simulink model "modelsim_cosimulation"  (R2021b)
settings: Solver=FixedStepDiscrete  StartTime=0.0  StopTime=4402*Ts  RelTol=1e-3
model workspace (MAT data in the model file):
  ErrMarginBits = 4
  Ts = 10
  inputdata.time = [0 10 20 30 40 50 60 70 80 90 100 110 ... (4402 elements, 4402x1)]
  inputdata.signals.values = embedded.fi
  inputdata.signals.values.DataType = 'Fixed'
  inputdata.signals.values.Scaling = 'BinaryPoint'
  inputdata.signals.values.Signed = 1
  inputdata.signals.values.WordLength = 12
  inputdata.signals.values.FixedExponent = 0
  inputdata.signals.values.SlopeAdjustmentFactor = 1
  inputdata.signals.values.Bias = 0
  inputdata.signals.values.DataTypeOverride = 'Inherit'
  inputdata.signals.values.intarray = [1 0 0 0 0 0 0 0 0 0 0 0 ... (4402 elements, 4402x1)]
  inputdata.signals.values.noverflows = 0
  inputdata.signals.values.nunderflows = 0
  inputdata.signals.values.maxlog = -1.79769313486e+308
  inputdata.signals.values.minlog = 1.79769313486e+308
  inputdata.signals.values.RoundingMethod = 'Round'
  inputdata.signals.values.OverflowAction = 'Saturate'
  inputdata.signals.values.ProductMode = 'FullPrecision'
  inputdata.signals.values.SumMode = 'FullPrecision'
  inputdata.signals.values.ProductWordLength = 32
  inputdata.signals.values.SumWordLength = 32
  inputdata.signals.values.MaxProductWordLength = 65535
  inputdata.signals.values.MaxSumWordLength = 65535
  inputdata.signals.values.ProductFractionLength = 30
  inputdata.signals.values.ProductFixedExponent = -30
  inputdata.signals.values.ProductSlope = 9.31322574615e-10
  inputdata.signals.values.ProductSlopeAdjustmentFactor = 1
  inputdata.signals.values.ProductBias = 0
  inputdata.signals.values.SumFractionLength = 30
  inputdata.signals.values.SumFixedExponent = -30
  inputdata.signals.values.SumSlope = 9.31322574615e-10
  inputdata.signals.values.SumSlopeAdjustmentFactor = 1
  inputdata.signals.values.SumBias = 0
  inputdata.signals.values.CastBeforeSum = 1
  inputdata.signals.values.DDGMaxProductWordLength = 65535
  inputdata.signals.values.DDGMaxSumWordLength = 65535
  inputdata.signals.values.DDGProductFixedExponent = -30
  inputdata.signals.values.DDGProductFractionLength = 30
  inputdata.signals.values.DDGProductWordLength = 32
  inputdata.signals.values.DDGSumFixedExponent = -30
  inputdata.signals.values.DDGSumFractionLength = 30
  inputdata.signals.values.DDGSumWordLength = 32
  inputdata.signals.values.DDGCastBeforeSum = 1
  inputdata.signals.values.DDGProductBias = 0
  inputdata.signals.values.DDGProductSlopeAdjustmentFactor = 1
  inputdata.signals.values.DDGSumBias = 0
  inputdata.signals.values.DDGSumSlopeAdjustmentFactor = 1
  inputdata.signals.values.DDGProductSlope = 9.31322574615e-10
  inputdata.signals.values.DDGSumSlope = 9.31322574615e-10
  inputdata.signals.values.Logging = 0
  inputdata.signals.values.fimathislocal = 1
  latency = 7
  resetdelay = 3
undefined symbols (not defined in the file or in its folder): clk, filter
libraries: simulink x1, modelsimlib x1
settings Model: Creator=caccolillo  LastModifiedBy=caccolillo

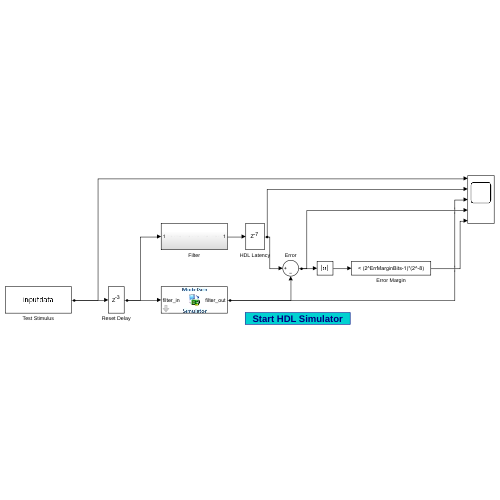
[thumbnail: Simulink's stored preview of the top-level diagram]
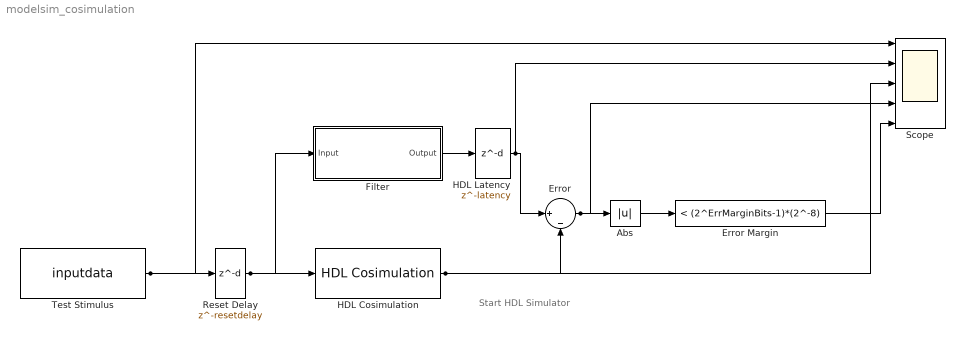
== system modelsim_cosimulation ==
  note: Start HDL Simulator
  Abs : Abs  SaturateOnIntegerOverflow=on
  Error : Sum  Inputs=||+|-  OutDataTypeStr=Inherit: Same as accumulator
  Error Margin : simulink/Logic and Bit Operations/Compare To Constant  relop=<  const=(2^ErrMarginBits-1)*(2^-8)  OutDataTypeStr=boolean
  Filter : Subsystem  Tag=FilterWizardSubSystem
      settings: ErrorFcn=dspFilterRealizedInBasicElemsAlgLoopErrFcnCallback
  HDL Cosimulation : modelsimlib/HDL Cosimulation  PortPaths=/filter/filter_in;/filter/filter_out  PortModes=[1 2 ]  PortTimes=[-1 Ts ]  PortSigns=[-1 1 ]  PortFracLengths=[0,8]  CommLocal=on  CommSharedMemory=on  CommPortNumber=4449  CommShowInfo=off  ClockPaths=filter/clk  ClockModes=[2 ]  ClockTimes=[10]  TclPreSimCommand=|  TclPostSimCommand=|  TimingMode=Tick  TimingScaleFactor=1  idxCellArray={'UNUSED_VAR'}  CosimBypass=Full Simulation  AllowDirectFeedthrough=on  ProductName=EDA Simulator Link MQ  RunAutoTimescale=off  HdlClocks=0  PreRunTime=0  PreRunTimeUnit=ns
      TclPreSimCommand=|
      | force /filter/clk_enable 0 0 ns, 1 32 ns;
      | force /filter/reset 1 0 ns, 0 22 ns;
      | puts -----------------------------------------
      | puts "Running Simulink Cosimulation block.";
      | puts [clock format [clock seconds]]
      TclPostSimCommand=|
      | force /filter/reset 1
      | puts [clock format [clock seconds]]
      settings: SourceProductBaseCode=ES
  HDL Latency : Delay  DelayLength=latency
  Reset Delay : Delay  DelayLength=resetdelay
  Scope : Scope  NumInputPorts=5
  Test Stimulus : FromWorkspace  VariableName=inputdata  SampleTime=Ts  Interpolate=off  OutputAfterFinalValue=Setting to zero
  wires:
  Test Stimulus/1 -> Reset Delay/1, Scope/1
  Reset Delay/1 -> HDL Cosimulation/1, Filter/1(Input)
  Filter/1(Output) -> HDL Latency/1
  HDL Latency/1 -> Error/1, Scope/2
  HDL Cosimulation/1 -> Error/2, Scope/3
  Error/1 -> Abs/1, Scope/4
  Abs/1 -> Error Margin/1
  Error Margin/1 -> Scope/5

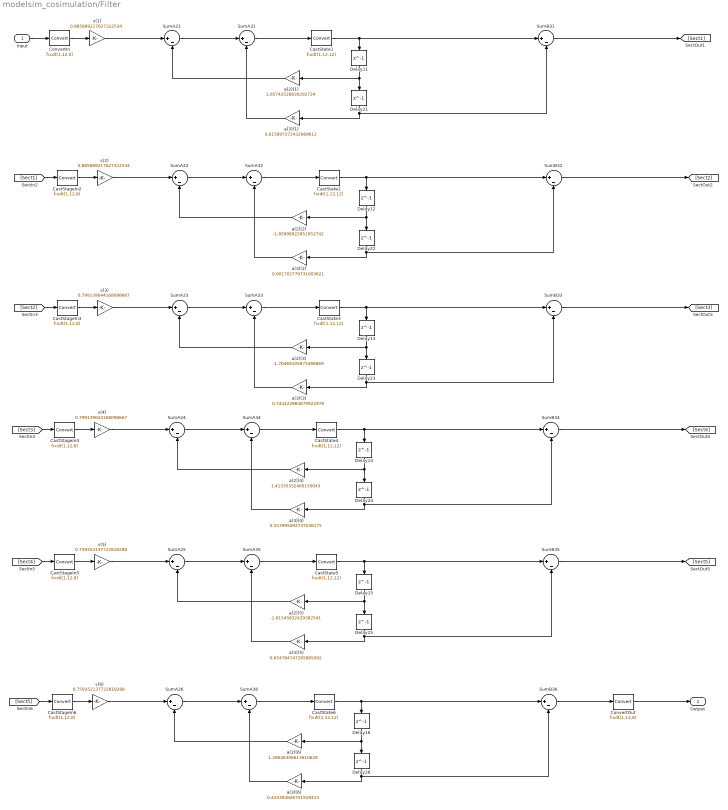
== system modelsim_cosimulation/Filter ==
  Input : Inport
  CastStageIn{2..6} (5 alike) : DataTypeConversion  OutDataTypeStr=fixdt(1,12,8)  RndMeth=Convergent  SaturateOnIntegerOverflow=on
  CastState{1..6} (6 alike) : DataTypeConversion  OutDataTypeStr=fixdt(1,12,12)  RndMeth=Convergent  SaturateOnIntegerOverflow=on
  ConvertIn : DataTypeConversion  OutDataTypeStr=fixdt(1,12,0)  RndMeth=Nearest  SaturateOnIntegerOverflow=on
  ConvertOut : DataTypeConversion  OutDataTypeStr=fixdt(1,12,8)  RndMeth=Convergent  SaturateOnIntegerOverflow=on
  Delay{11..16,21..26} (12 alike) : Delay  DelayLength=1  InitialCondition=0
  SumA{21..26,31..36} (12 alike) : Sum  Inputs=|+-  AccumDataTypeStr=fixdt(1,40,22)  OutDataTypeStr=fixdt(1,40,22)  RndMeth=Convergent  SaturateOnIntegerOverflow=on
  SumB{31..36} (6 alike) : Sum  Inputs=|+-  AccumDataTypeStr=fixdt(1,40,22)  OutDataTypeStr=fixdt(1,40,22)  RndMeth=Convergent  SaturateOnIntegerOverflow=on
  a(2)(1) : Gain  Gain=1.65742528830292724  ParamDataTypeStr=fixdt(1,12,10)  OutDataTypeStr=fixdt(1,24,22)  RndMeth=Convergent  SaturateOnIntegerOverflow=on
  a(2)(2) : Gain  Gain=-1.85998922851952742  ParamDataTypeStr=fixdt(1,12,10)  OutDataTypeStr=fixdt(1,24,22)  RndMeth=Convergent  SaturateOnIntegerOverflow=on
  a(2)(3) : Gain  Gain=-1.70469105875488869  ParamDataTypeStr=fixdt(1,12,10)  OutDataTypeStr=fixdt(1,24,22)  RndMeth=Convergent  SaturateOnIntegerOverflow=on
  a(2)(4) : Gain  Gain=1.41335332460150043  ParamDataTypeStr=fixdt(1,12,10)  OutDataTypeStr=fixdt(1,24,22)  RndMeth=Convergent  SaturateOnIntegerOverflow=on
  a(2)(5) : Gain  Gain=-1.61545832429382541  ParamDataTypeStr=fixdt(1,12,10)  OutDataTypeStr=fixdt(1,24,22)  RndMeth=Convergent  SaturateOnIntegerOverflow=on
  a(2)(6) : Gain  Gain=1.28646306613610628  ParamDataTypeStr=fixdt(1,12,10)  OutDataTypeStr=fixdt(1,24,22)  RndMeth=Convergent  SaturateOnIntegerOverflow=on
  a(3)(1) : Gain  Gain=0.815897372432069612  ParamDataTypeStr=fixdt(1,12,10)  OutDataTypeStr=fixdt(1,24,22)  RndMeth=Convergent  SaturateOnIntegerOverflow=on
  a(3)(2) : Gain  Gain=0.901702779731603621  ParamDataTypeStr=fixdt(1,12,10)  OutDataTypeStr=fixdt(1,24,22)  RndMeth=Convergent  SaturateOnIntegerOverflow=on
  a(3)(3) : Gain  Gain=0.744422984879922978  ParamDataTypeStr=fixdt(1,12,10)  OutDataTypeStr=fixdt(1,24,22)  RndMeth=Convergent  SaturateOnIntegerOverflow=on
  a(3)(4) : Gain  Gain=0.553995092737038175  ParamDataTypeStr=fixdt(1,12,10)  OutDataTypeStr=fixdt(1,24,22)  RndMeth=Convergent  SaturateOnIntegerOverflow=on
  a(3)(5) : Gain  Gain=0.654784747265885092  ParamDataTypeStr=fixdt(1,12,10)  OutDataTypeStr=fixdt(1,24,22)  RndMeth=Convergent  SaturateOnIntegerOverflow=on
  a(3)(6) : Gain  Gain=0.420394826751919415  ParamDataTypeStr=fixdt(1,12,10)  OutDataTypeStr=fixdt(1,24,22)  RndMeth=Convergent  SaturateOnIntegerOverflow=on
  s(1) : Gain  Gain=0.885889217627322534  ParamDataTypeStr=fixdt(1,12,11)  OutDataTypeStr=fixdt(1,12,7)  RndMeth=Convergent  SaturateOnIntegerOverflow=on
  s(2) : Gain  Gain=0.885889217627322534  ParamDataTypeStr=fixdt(1,12,11)  OutDataTypeStr=fixdt(1,12,7)  RndMeth=Convergent  SaturateOnIntegerOverflow=on
  s(3) : Gain  Gain=0.799139044168098667  ParamDataTypeStr=fixdt(1,12,11)  OutDataTypeStr=fixdt(1,12,7)  RndMeth=Convergent  SaturateOnIntegerOverflow=on
  s(4) : Gain  Gain=0.799139044168098667  ParamDataTypeStr=fixdt(1,12,11)  OutDataTypeStr=fixdt(1,12,7)  RndMeth=Convergent  SaturateOnIntegerOverflow=on
  s(5) : Gain  Gain=0.759352137722818288  ParamDataTypeStr=fixdt(1,12,11)  OutDataTypeStr=fixdt(1,12,7)  RndMeth=Convergent  SaturateOnIntegerOverflow=on
  s(6) : Gain  Gain=0.759352137722818288  ParamDataTypeStr=fixdt(1,12,11)  OutDataTypeStr=fixdt(1,12,7)  RndMeth=Convergent  SaturateOnIntegerOverflow=on
  Output : Outport
  wires:
  Input/1 -> ConvertIn/1
  s(1)/1 -> SumA21/1
  SumA21/1 -> SumA31/1
  SumA31/1 -> CastState1/1
  CastState1/1 -> SumB31/1, Delay11/1
  SumB31/1 -> [Sect1]
  a(2)(1)/1 -> SumA21/2
  Delay11/1 -> a(2)(1)/1, Delay21/1
  a(3)(1)/1 -> SumA31/2
  Delay21/1 -> a(3)(1)/1, SumB31/2
  ConvertIn/1 -> s(1)/1
  [Sect1] -> CastStageIn2/1
  s(2)/1 -> SumA22/1
  SumA22/1 -> SumA32/1
  SumA32/1 -> CastState2/1
  CastState2/1 -> SumB32/1, Delay12/1
  SumB32/1 -> [Sect2]
  a(2)(2)/1 -> SumA22/2
  Delay12/1 -> a(2)(2)/1, Delay22/1
  a(3)(2)/1 -> SumA32/2
  Delay22/1 -> a(3)(2)/1, SumB32/2
  CastStageIn2/1 -> s(2)/1
  [Sect2] -> CastStageIn3/1
  s(3)/1 -> SumA23/1
  SumA23/1 -> SumA33/1
  SumA33/1 -> CastState3/1
  CastState3/1 -> SumB33/1, Delay13/1
  SumB33/1 -> [Sect3]
  a(2)(3)/1 -> SumA23/2
  Delay13/1 -> a(2)(3)/1, Delay23/1
  a(3)(3)/1 -> SumA33/2
  Delay23/1 -> a(3)(3)/1, SumB33/2
  CastStageIn3/1 -> s(3)/1
  [Sect3] -> CastStageIn4/1
  s(4)/1 -> SumA24/1
  SumA24/1 -> SumA34/1
  SumA34/1 -> CastState4/1
  CastState4/1 -> SumB34/1, Delay14/1
  SumB34/1 -> [Sect4]
  a(2)(4)/1 -> SumA24/2
  Delay14/1 -> a(2)(4)/1, Delay24/1
  a(3)(4)/1 -> SumA34/2
  Delay24/1 -> a(3)(4)/1, SumB34/2
  CastStageIn4/1 -> s(4)/1
  [Sect4] -> CastStageIn5/1
  s(5)/1 -> SumA25/1
  SumA25/1 -> SumA35/1
  SumA35/1 -> CastState5/1
  CastState5/1 -> SumB35/1, Delay15/1
  SumB35/1 -> [Sect5]
  a(2)(5)/1 -> SumA25/2
  Delay15/1 -> a(2)(5)/1, Delay25/1
  a(3)(5)/1 -> SumA35/2
  Delay25/1 -> a(3)(5)/1, SumB35/2
  CastStageIn5/1 -> s(5)/1
  [Sect5] -> CastStageIn6/1
  s(6)/1 -> SumA26/1
  SumA26/1 -> SumA36/1
  SumA36/1 -> CastState6/1
  CastState6/1 -> SumB36/1, Delay16/1
  SumB36/1 -> ConvertOut/1
  a(2)(6)/1 -> SumA26/2
  Delay16/1 -> a(2)(6)/1, Delay26/1
  a(3)(6)/1 -> SumA36/2
  Delay26/1 -> a(3)(6)/1, SumB36/2
  ConvertOut/1 -> Output/1
  CastStageIn6/1 -> s(6)/1
